simulink model "sldvdemo_thrustrvs_int_original"  (R2020a)
settings: Solver=FixedStepDiscrete  StartTime=0.0  StopTime=10.0  FixedStep=.1  RelTol=1e-3  EnableMultiTasking=on
PreLoadFcn:
  | load sldvdemo_thrust_reverse_bus.mat
Description:
  | Thrust Reverser Fixed
settings Model: Creator=The MathWorks, Inc.  LastModifiedBy=patcanny
settings DataIOCC: ExternalInput=testdata  LimitDataPoints=on  SaveFormat=Array  ReturnWorkspaceOutputs=off
settings OptimizationCC: DefaultParameterBehavior=Inlined  ExpressionDepthLimit=2147483647  InitFltsAndDblsToZero=on  LifeSpan=1  EfficientTunableParamExpr=on
settings DebuggingCC: UnderspecifiedInitializationDetection=Classic  MergeDetectMultiDrivingBlocksExec=none  SolverPrmCheckMsg=warning  FcnCallInpInsideContextMsg=warning  AllowSymbolicDim=off  StateNameClashWarn=warning  SymbolicDimsDataTypeCodeGenerationDiagnostic=none  SFUnexpectedBacktrackingDiag=warning  SFNoUnconditionalDefaultTransitionDiag=warning  SFExecutionAtInitializationDiag=none  ArithmeticOperatorsInVariantConditions=warning
settings HardwareCC: ProdBitPerPointer=32  ProdBitPerSizeT=32  ProdBitPerPtrDiffT=32  ProdLargestAtomicFloat=None  ProdIntDivRoundTo=Undefined  ProdEndianess=Unspecified  ProdWordSize=32  ProdHWDeviceType=32-bit Generic
settings ModelReferenceCC: PropagateSignalLabelsOutOfModel=off
settings SFSimCC: SimUseLocalCustomCode=off  SimParseCustomCode=off  MATLABDynamicMemAlloc=off  CustomCodeUndefinedFunction=UseInterfaceOnly
settings RTWCC: Description=Real-Time Workshop Embedded Coder (no auto configuration)  SystemTargetFile=ert.tlc  GenCodeOnly=on  TemplateMakefile=ert_default_tmf  RTWUseLocalCustomCode=off
settings CodeAppCC: IgnoreCustomStorageClasses=off  CustomSymbolStrType=$N$R$M  CustomSymbolStrModelFcn=$N  StateflowObjectComments=on  InternalIdentifier=Classic
settings ERTTargetCC: MultiwordLength=2048  GenerateSampleERTMain=on  InlinedParameterPlacement=NonHierarchical  ERTCustomFileTemplate=example_file_process.tlc  ConvertIfToSwitch=off  SuppressUnreachableDefaultCases=off
settings ConfigComp: DVMaxProcessTime=600  DVParameters=on  DVModelCoverageObjectives=MCDC  DVMaxTestCaseSteps=500  DVTestSuiteOptimization=Auto  DVDetectActiveLogic=on  DVRebuildModelRepresentation=Always

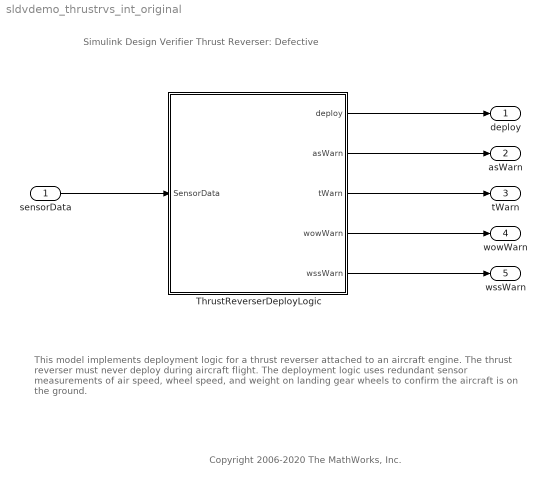
== system sldvdemo_thrustrvs_int_original ==
  note: Copyright 2006-2020 The MathWorks, Inc.
  note: This model implements deployment logic for a thrust reverser attached to an aircraft engine.
      | The thrust reverser must never deploy during aircraft flight.  The deployment logic uses redundant
      | sensor measurements of air speed, wheel speed, and weight on landing gear wheels to confirm
      | the aircraft is on the ground.
  note: Simulink Design Verifier Thrust Reverser: Defective
  sensorData : Inport  OutDataTypeStr=Bus: sldvThrustReverseBus
  ThrustReverserDeployLogic : Stateflow chart  TreatAsAtomicUnit=on
  deploy : Outport  OutDataTypeStr=boolean  PortDimensions=1  VectorParamsAs1DForOutWhenUnconnected=off
  asWarn : Outport  Port=2  OutDataTypeStr=boolean  PortDimensions=1  VectorParamsAs1DForOutWhenUnconnected=off
  tWarn : Outport  Port=3  OutDataTypeStr=boolean  PortDimensions=1  VectorParamsAs1DForOutWhenUnconnected=off
  wowWarn : Outport  Port=4  OutDataTypeStr=boolean  PortDimensions=1  VectorParamsAs1DForOutWhenUnconnected=off
  wssWarn : Outport  Port=5  OutDataTypeStr=boolean  PortDimensions=1  VectorParamsAs1DForOutWhenUnconnected=off
  wires:
  sensorData/1 -> ThrustReverserDeployLogic/1(SensorData)
  ThrustReverserDeployLogic/1(deploy) -> deploy/1
  ThrustReverserDeployLogic/2(asWarn) -> asWarn/1
  ThrustReverserDeployLogic/3(tWarn) -> tWarn/1
  ThrustReverserDeployLogic/4(wowWarn) -> wowWarn/1
  ThrustReverserDeployLogic/5(wssWarn) -> wssWarn/1

== stateflow chart sldvdemo_thrustrvs_int_original/ThrustReverserDeployLogic ==
  state thrustReversers [parallel]
    settings: executionOrder=1
    state undeployed
      en:deploy=0;
    state deployed
      en:deploy=1;
    (default) -> undeployed
    undeployed -> deployed : [(onGround(SensorData.wowSensors) +...
        |  isRolling(SensorData.wheelSpeedSensors) +...
        |  airspeedOK(SensorData.airSpeedSensors) >=2) &&...
        |  throttleOK(SensorData.throttlePositions)]
    deployed -> undeployed : [!throttleOK(SensorData.throttlePositions)]
  state og = onGround(ww) [function]
    (default) -> (junction 279)
    (junction 279) -> (junction 281) : {
        | /* 1st weight on wheel sensor for left gear */
        | aVarTruthTableCondition_1 = (ww[1]);
        | }
    (junction 281) -> (junction 283) : {
        | /* 2nd weight on wheel sensor for left gear */
        | aVarTruthTableCondition_2 = (ww[2]);
        | }
    (junction 283) -> (junction 285) : {
        | /* 1st weight on wheel sensor for right gear */
        | aVarTruthTableCondition_3 = (ww[3]);
        | }
    (junction 285) -> (junction 287) : {
        | /* 2nd weight on wheel sensor for right gear */
        | aVarTruthTableCondition_4 = (ww[4]);
        | }
    (junction 287) -> (junction 289) [order 1] : [aVarTruthTableCondition_1 && aVarTruthTableCondition_2 && aVarTruthTableCondition_3 && aVarTruthTableCondition_4]
    (junction 289) -> (junction 291) : {
        | /* Wheels are on the ground */
        | og = 1;
        | }
    (junction 287) -> (junction 293) [order 2]
    (junction 293) -> (junction 295) [order 1] : [!aVarTruthTableCondition_1 && !aVarTruthTableCondition_2 && !aVarTruthTableCondition_3 && !aVarTruthTableCondition_4]
    (junction 295) -> (junction 297) : {
        | /* Wheels are not on the ground */
        | og = 0;
        | }
    (junction 293) -> (junction 299) [order 2]
    (junction 299) -> (junction 301) [order 1] : [aVarTruthTableCondition_1 && aVarTruthTableCondition_2]
    (junction 301) -> (junction 303) : {
        | /* Wheels are on the ground */
        | og = 1;
        | }
    (junction 303) -> (junction 305) : {
        | /* Broadcast warning that sensors do not all agree */
        | send(wowE,warnings)
        | }
    (junction 299) -> (junction 307) [order 2]
    (junction 307) -> (junction 309) [order 1] : [aVarTruthTableCondition_3 && aVarTruthTableCondition_4]
    (junction 309) -> (junction 311) : {
        | /* Wheels are on the ground */
        | og = 1;
        | }
    (junction 311) -> (junction 313) : {
        | /* Broadcast warning that sensors do not all agree */
        | send(wowE,warnings)
        | }
    (junction 307) -> (junction 315) [order 2]
    (junction 315) -> (junction 317) : /* Default */
    (junction 317) -> (junction 319) : {
        | /* Wheels are not on the ground */
        | og = 0;
        | }
    (junction 319) -> (junction 321) : {
        | /* Broadcast warning that sensors do not all agree */
        | send(wowE,warnings)
        | }
  state ir=isRolling(ws) [function]
    note: WST = Wheel Speed Threshold
    note: I assume that a "bad" wheel speed
        | sensor gives a value of 0...?
    (default) -> (junction 100)
    (junction 100) -> (junction 117) [order 2] : [ws[1]<WST && ws[2]<WST]
    (junction 100) -> (junction 116) [order 1] : [ws[1]>=WST && ws[2]>=WST]
    (junction 117) -> (junction 118)
    (junction 116) -> (junction 121)
    (junction 100) -> (junction 119) [order 3] : {send(wssE,warnings)}
    (junction 121) -> (junction 119)
    (junction 119) -> (junction 122) : {ir=1;}
    (junction 118) -> (junction 122) : {ir=0;}
  state warnings [parallel]
    settings: executionOrder=2
    state wsSensors [parallel]
      settings: executionOrder=1
      state agree
        en:wssWarn=0;
      state notAgree
        en:wssWarn=1;
      (default) -> warnings.wsSensors.agree
      warnings.wsSensors.agree -> warnings.wsSensors.notAgree : wssE
    state wowSensors [parallel]
      settings: executionOrder=2
      state agree
        en:wowWarn=0;
      state notAgree
        en:wowWarn=1;
      (default) -> warnings.wowSensors.agree
      warnings.wowSensors.agree -> warnings.wowSensors.notAgree : wowE
    state airspeedSensors [parallel]
      settings: executionOrder=3
      state agree
        en:asWarn=0;
      state notAgree
        en:asWarn=1;
      (default) -> warnings.airspeedSensors.agree
      warnings.airspeedSensors.agree -> warnings.airspeedSensors.notAgree : asE
    state throttleSensors [parallel]
      settings: executionOrder=4
      state agree
        en:tWarn=0;
      state notAgree
        en:tWarn=1;
      (default) -> warnings.throttleSensors.agree
      warnings.throttleSensors.agree -> warnings.throttleSensors.notAgree : tE
  state aok=airspeedOK(as) [function]
    (default) -> (junction 101)
    (junction 101) -> (junction 106) [order 2] : {send(asE,warnings)}
    (junction 101) -> (junction 112) [order 1] : // within 5 knots of each other
        | [closeEnough(as[1],as[2],5)]
    (junction 112) -> (junction 113) [order 1] : //if the average is less than the threshold
        | [((as[1]+as[2])/2)<maxAS]
    (junction 112) -> (junction 106) [order 2]
    (junction 113) -> (junction 120)
    (junction 106) -> (junction 105) : {aok=0;}
    (junction 120) -> (junction 105) : {aok=1;}
  state tok=throttleOK(ts) [function]
    note: {send(tE,warnings)}
    note: Flag set to sensor reading
    (default) -> (junction 127)
    (junction 127) -> (junction 125) [order 3] : {var=0;}
    (junction 125) -> (junction 129) [order 2] : {send(tE,warnings)}
    (junction 127) -> (junction 126) [order 1] : [ts[1]>=thT &&...
        | ts[2]>=thT &&...
        | ts[3]>=thT &&...
        | ts[4]>=thT]
    (junction 127) -> (junction 126) [order 2] : [ts[1]<thT &&...
        |  ts[2]<thT &&...
        |  ts[3]<thT &&...
        |  ts[4]<thT]
    (junction 125) -> (junction 124) [order 1] : [closeEnough(ts[1],ts[2],1)]
    (junction 124) -> (junction 123) [order 1] : [(ts[1]+ts[2])/2<thT]
    (junction 124) -> (junction 129) [order 2]
    (junction 123) -> (junction 130) : {var++;}
    (junction 130) -> (junction 129)
    (junction 129) -> (junction 102) [order 2] : {send(tE,warnings)}
    (junction 129) -> (junction 132) [order 1] : [closeEnough(ts[3],ts[4],1)]
    (junction 126) -> (junction 128) : {tok=(ts[1]<thT);}
    (junction 132) -> (junction 131) [order 1] : [(ts[3]+ts[4])/2<thT]
    (junction 132) -> (junction 133) [order 2] : {var=0;}
    (junction 131) -> (junction 134) : {var++;}
    (junction 134) -> (junction 133)
    (junction 133) -> (junction 102)
    (junction 102) -> (junction 135) : {tok=(var>1);}
    (junction 128) -> (junction 135)
  data: og function_output uint8; ww function_input boolean size=4; aVarTruthTableCondition_1 temporary boolean =0; aVarTruthTableCondition_2 temporary boolean =0; aVarTruthTableCondition_3 temporary boolean =0; aVarTruthTableCondition_4 temporary boolean =0; ws function_input int16 size=2; ir function_output uint8; as function_input int16 size=2; aok function_output boolean; ts function_input int8 size=4; tok function_output boolean; n1 function_input int16; n2 function_input int16; tol function_input int16; isclose function_output int8; deploy output boolean size=1; SensorData input sldvThrustReverseBus size=1; var local int16; WST constant int16 =10; maxAS constant int16 size=1 =150; thT constant int8 size=1 =-1; asWarn output boolean; tWarn output boolean; wowWarn output boolean; wssWarn output boolean
  data aVarTruthTableCondition_1 settings: description=1st weight on wheel sensor for left gear
  data aVarTruthTableCondition_2 settings: description=2nd weight on wheel sensor for left gear
  data aVarTruthTableCondition_3 settings: description=1st weight on wheel sensor for right gear
  data aVarTruthTableCondition_4 settings: description=2nd weight on wheel sensor for right gear
  events: asE local EITHER_EDGE_EVENT; tE local EITHER_EDGE_EVENT; wowE local EITHER_EDGE_EVENT; wssE local EITHER_EDGE_EVENT
  function isclose = closeEnough(n1,n2,tol):
    | function isclose = closeEnough(n1,n2,tol)
    |  if abs(n1-n2) <= tol
    |      isclose=int8(1);
    |  else
    |      isclose=int8(0);
    |  end
